simulink model "MicroADAPCPU1"  (R2024a)
settings: Solver=FixedStepAuto  StartTime=0.0  StopTime=Inf  RelTol=1e-3  EnableMultiTasking=on
PreLoadFcn:
  | %Condiciones iniciales
  | id0=single(0);
  | iq0=single(0);
  | w0=single(0);
  | Thetha0=single(0);
  | deltars=0;
  | deltaLd=0;
  | deltaLq=0;
  | deltaphi=0;
  | 
  | %Parametros Axel;
  | Rs=single(1.1); %Ohms
  | L=single(0.00372);
  | Ld=L; %Henrry
  | Lq=L; %Henrry
  | Jm=single(0.00023998); %Kg m2
  | Rm=single(0.0006738); %Nm s
  | rm=Rm;
  | phi=single(0.1099); %Wb
  | %0.0582
  | np=single(8);
values from neighbouring files (symbols this model uses):
  target = mcb_SetProcessorDetails('F28379D',PWM_frequency)    [Para_Motor_Micro.m]
  Ts_com = 2*1*Ts    (= 6e-05)    [Para_Motor_Micro.m]
undefined symbols (not defined in the file or in its folder): C28x, CPU1, CPU2, DiscIntNeverNeededParam, Down, GPTRIP1SEL, GPTRIP2SEL, inverter, PWM_Counter_PeriodVel, TZ1, TZ2, Up
libraries: c2802xlib x12, mcbcontrolslib x9, c2837xDlib x8, simulink x4, mcbpositiondecoderlib x3, c280xlib x3, svdutilitieslib x2, eeTransforms x1, c2000lib x1
(part 1 of 2)
settings Model: ExtModeTrigDuration=8  Creator=axel_  LastModifiedBy=axel_
settings SolverCC: AutoInsertRateTranBlk=on
settings OptimizationCC: DefaultParameterBehavior=Inlined  DefaultUnderspecifiedDataType=single  EnhancedBackFolding=on  PassReuseOutputArgsAs=Individual arguments  MaxStackSize=1024  OptimizeBlockOrder=speed  DifferentSizesBufferReuse=on  OptimizationCustomize=off  DenormalBehavior=FlushToZero  EfficientTunableParamExpr=on
settings DebuggingCC: MultiTaskDSMMsg=none  ParameterPrecisionLossMsg=none  ParameterTunabilityLossMsg=error
settings HardwareCC: ProdBitPerChar=16  ProdBitPerInt=16  ProdBitPerPointer=32  ProdBitPerSizeT=32  ProdBitPerPtrDiffT=32  ProdLargestAtomicInteger=Integer  ProdLargestAtomicFloat=None  ProdWordSize=16  ProdHWDeviceType=Texas Instruments->C2000
settings ModelReferenceCC: ModelReferenceNumInstancesAllowed=Single
settings SFSimCC: MATLABDynamicMemAlloc=off
settings RTWCC: Description=Embedded Coder  SystemTargetFile=ert.tlc  HardwareBoard=TI Delfino F2837xD  TemplateMakefile=ert_default_tmf  Toolchain=Texas Instruments Code Composer Studio (C2000)  GPUComputeCapability=3.5
settings CodeAppCC: ForceParamTrailComments=on  IgnoreCustomStorageClasses=off  OperatorAnnotations=on  SimulinkDataObjDesc=on  SFDataObjDesc=on  InsertBlockDesc=on
settings ERTTargetCC: CodeReplacementLibrary=TI C28x  ExtModeTransport=4  ExtModeStaticAlloc=on  ExtModeAutomaticAllocSize=off  ExtModeStaticAllocSize=10000  ExtModeMexFile=ext_xcp  ExtModeIntrfLevel=Level2 - Open  InlinedParameterPlacement=NonHierarchical

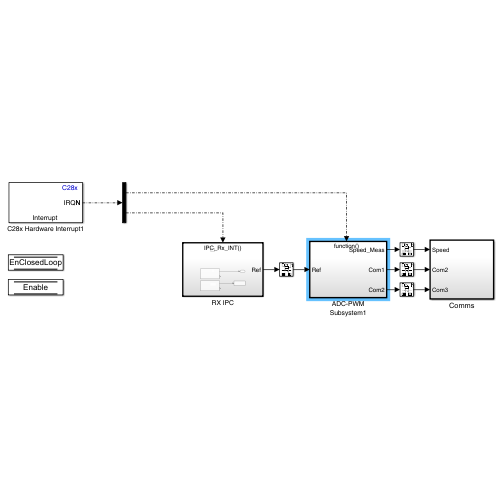
[thumbnail: Simulink's stored preview of the top-level diagram]
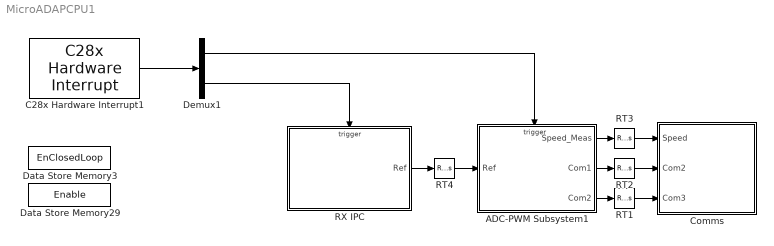
== system MicroADAPCPU1 ==
  ADC-PWM Subsystem1 : Subsystem  TreatAsAtomicUnit=on
  C28x Hardware Interrupt1 : c2000lib/Scheduling/C28x Hardware Interrupt  irqnumbers=[1 1 ]  pienumbers=[1 15 ]  irqpriorities=[30 40 ]  irqpreempts="[1   0  ]"  showinput=off  dspchiptype=C280X
  Comms : Subsystem  TreatAsAtomicUnit=on  SystemSampleTime=Ts_com
  Data Store Memory29 : DataStoreMemory  DataStoreName=Enable  ShowAdditionalParam=off  OutDataTypeStr=boolean
  Data Store Memory3 : DataStoreMemory  DataStoreName=EnClosedLoop  ShowAdditionalParam=off  OutDataTypeStr=boolean
  Demux1 : Demux  Outputs=2
  RT{1..4} (4 alike) : RateTransition  Deterministic=off
  RX IPC : Subsystem
  wires:
  C28x Hardware Interrupt1/1 -> Demux1/1
  Demux1/1 -> ADC-PWM Subsystem1/Trigger
  ADC-PWM Subsystem1/1(Speed_Meas) -> RT3/1
  ADC-PWM Subsystem1/2(Com1) -> RT2/1
  ADC-PWM Subsystem1/3(Com2) -> RT1/1
  RT3/1 -> Comms/1(Speed)
  RT2/1 -> Comms/2(Com2)
  RT1/1 -> Comms/3(Com3)
  RX IPC/1(Ref) -> RT4/1
  Demux1/2 -> RX IPC/Trigger
  RT4/1 -> ADC-PWM Subsystem1/1(Ref)

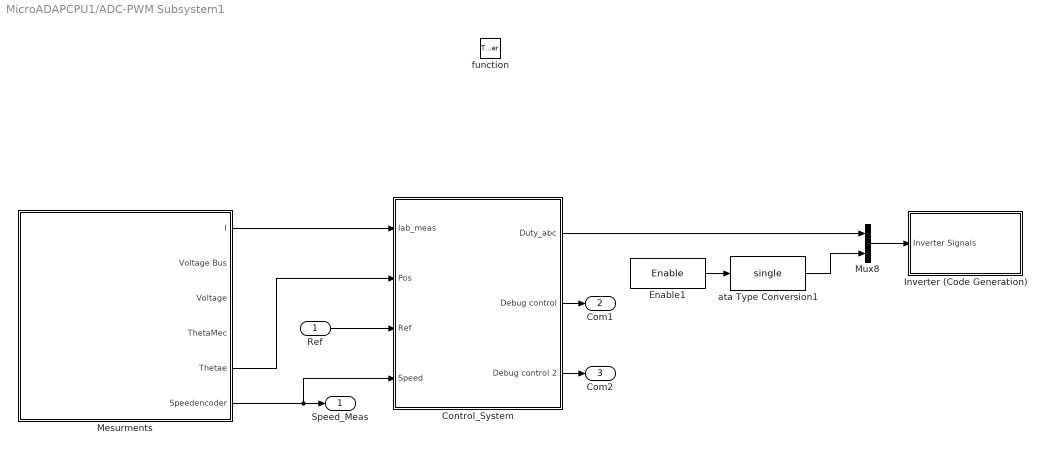
== system MicroADAPCPU1/ADC-PWM Subsystem1 ==
  Ref : Inport
  function : TriggerPort  TriggerType=function-call  VariantControl=Variant  OutputDataType=int8
  Control_System : Subsystem  SystemSampleTime=5e-5
  Enable1 : DataStoreRead  DataStoreName=Enable  IndexOptions=Index vector (dialog)  Indices=1  OutputSizes=1
  Inverter (Code Generation) : Subsystem
  Mesurments : Subsystem
  Mux8 : Mux  Inputs=2
  ata Type Conversion1 : DataTypeConversion  OutDataTypeStr=single  SaturateOnIntegerOverflow=off  RndMeth=Floor
  Speed_Meas : Outport
  Com1 : Outport  Port=2
  Com2 : Outport  Port=3
  wires:
  Ref/1 -> Control_System/3(Ref)
  Mesurments/1(I) -> Control_System/1(Iab_meas)
  Mesurments/6(Speedencoder) -> Control_System/4(Speed), Speed_Meas/1
  Mesurments/5(Thetae) -> Control_System/2(Pos)
  ata Type Conversion1/1 -> Mux8/2
  Control_System/1(Duty_abc) -> Mux8/1
  Enable1/1 -> ata Type Conversion1/1
  Mux8/1 -> Inverter (Code Generation)/1(Inverter Signals)
  Control_System/2(Debug control) -> Com1/1
  Control_System/3(Debug control 2) -> Com2/1

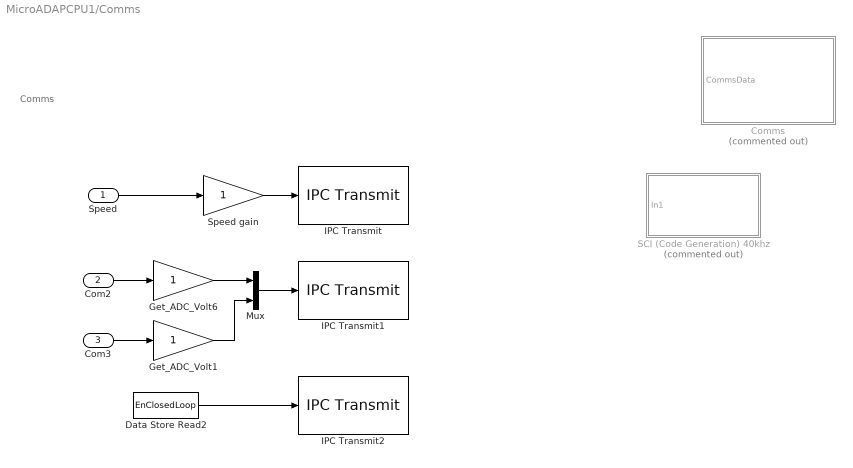
== system MicroADAPCPU1/Comms ==
  note: Comms
  Speed : Inport
  Com2 : Inport  Port=2
  Com3 : Inport  Port=3
  Comms : Subsystem  Commented=on  SystemSampleTime=5e-5
  Data Store Read2 : DataStoreRead  DataStoreName=EnClosedLoop  IndexOptions=Index vector (dialog)  Indices=1  OutputSizes=1
  Get_ADC_Volt1 : Gain  OutDataTypeStr=single  RndMeth=Simplest
  Get_ADC_Volt6 : Gain  OutDataTypeStr=single  RndMeth=Simplest
  IPC Transmit : c2837xDlib/IPC Transmit  blkParamProc=F2837x  SelectDestination=C28x (CPU1/CPU2)  SelectChannel=0  EnableBlocking=off
  IPC Transmit1 : c2837xDlib/IPC Transmit  blkParamProc=F2837x  SelectDestination=C28x (CPU1/CPU2)  SelectChannel=1  EnableBlocking=off
  IPC Transmit2 : c2837xDlib/IPC Transmit  blkParamProc=F2837x  SelectDestination=C28x (CPU1/CPU2)  SelectChannel=4  EnableBlocking=off
  Mux : Mux  Inputs=2
  SCI (Code Generation) 40khz : Subsystem  Commented=on
  Speed gain : Gain  OutDataTypeStr=single  RndMeth=Simplest
  wires:
  Speed/1 -> Speed gain/1
  Com2/1 -> Get_ADC_Volt6/1
  Speed gain/1 -> IPC Transmit/1
  Com3/1 -> Get_ADC_Volt1/1
  Get_ADC_Volt6/1 -> Mux/1
  Get_ADC_Volt1/1 -> Mux/2
  Mux/1 -> IPC Transmit1/1
  Data Store Read2/1 -> IPC Transmit2/1

== system MicroADAPCPU1/RX IPC ==
  note: Data 1
  note: Te
  IPC_Rx_INT : TriggerPort  TriggerType=function-call  VariantControl=Variant
  Data Store Write : DataStoreWrite  DataStoreName=Enable  IndexOptions=Index vector (dialog)  Indices=1  OutputSizes=1
  IPC Receive1 : c2837xDlib/IPC Receive  blkParamProc=F2837x  SelectSource=C28x (CPU1/CPU2)  SelectChannel=2  DataType=single  DataLength=1  EnableBlocking=off  SampleTime=-1
  IPC Receive2 : c2837xDlib/IPC Receive  blkParamProc=F2837x  SelectSource=C28x (CPU1/CPU2)  SelectChannel=3  DataType=boolean  DataLength=1  EnableBlocking=off  SampleTime=-1
  Ref : Outport
  wires:
  IPC Receive1/1 -> Ref/1
  IPC Receive2/1 -> Data Store Write/1

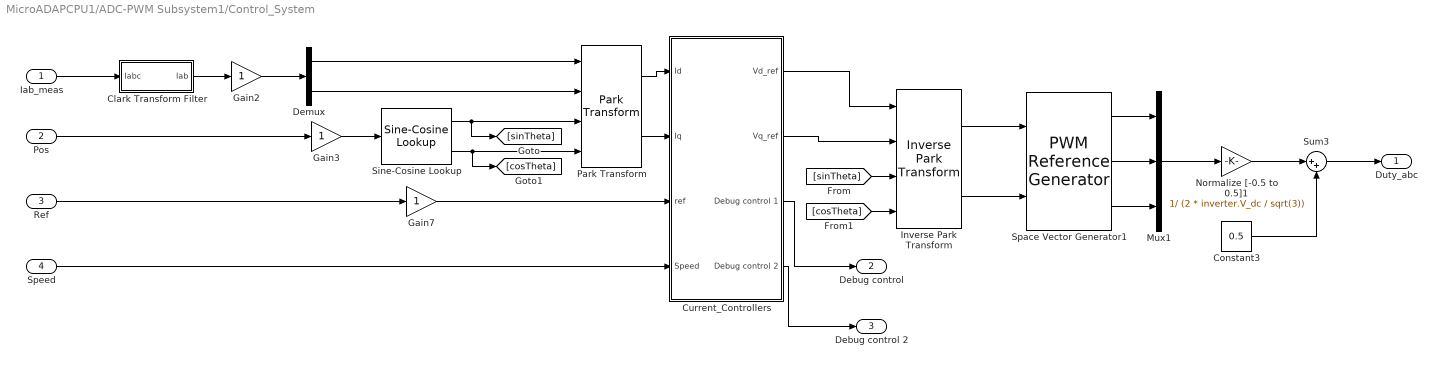
== system MicroADAPCPU1/ADC-PWM Subsystem1/Control_System ==
  Iab_meas : Inport
  Pos : Inport  Port=2
  Ref : Inport  Port=3
  Speed : Inport  Port=4
  Clark Transform Filter : Subsystem
  Constant3 : Constant  Value=0.5  OutDataTypeStr=dataType  SampleTime=-1
  Current_Controllers : Subsystem
  Demux : Demux  Outputs=2
  Gain2 : Gain  OutDataTypeStr=single
  Gain3 : Gain  OutDataTypeStr=single
  Gain7 : Gain
  Inverse Park Transform : mcbcontrolslib/Inverse Park Transform  PhaseInput=Two inputs  AxisAlignment=D-axis  ThetaInput=Sine and Cosine electrical position  AngleInput=Per-unit  N_points=1024
  Mux1 : Mux  Inputs=3
  Normalize [-0.5 to 0.5]1 : Gain  Gain=1/ (2 * inverter.V_dc / sqrt(3))  RndMeth=Simplest  OutDataTypeStr=Inherit: Same as input
  Park Transform : mcbcontrolslib/Park Transform  PhaseInput=Two inputs  AxisAlignment=D-axis  ThetaInput=Sine and Cosine electrical position  AngleInput=Per-unit  N_points=1024
  Sine-Cosine Lookup : mcbcontrolslib/Sine-Cosine Lookup  AngleInput=Radians  N_points=1024  DatatypeInput=Inherit from input  Datatype=single
  Space Vector Generator1 : mcbcontrolslib/PWM Reference Generator  inSignal=Valphabeta  modType=SPWM: sinusoidal PWM
  Sum3 : Sum  Inputs=|++
  Duty_abc : Outport  VectorParamsAs1DForOutWhenUnconnected=off
  Debug control : Outport  Port=2
  Debug control 2 : Outport  Port=3
  wires:
  Gain3/1 -> Sine-Cosine Lookup/1
  Ref/1 -> Gain7/1
  Sine-Cosine Lookup/2 -> Park Transform/4, [cosTheta]
  Park Transform/1 -> Current_Controllers/1(Id)
  Gain2/1 -> Demux/1
  Demux/1 -> Park Transform/1
  Current_Controllers/2(Vq_ref) -> Inverse Park Transform/2
  Pos/1 -> Gain3/1
  [sinTheta] -> Inverse Park Transform/3
  Park Transform/2 -> Current_Controllers/2(Iq)
  Gain7/1 -> Current_Controllers/3(ref)
  [cosTheta] -> Inverse Park Transform/4
  Inverse Park Transform/1 -> Space Vector Generator1/1
  Inverse Park Transform/2 -> Space Vector Generator1/2
  Current_Controllers/1(Vd_ref) -> Inverse Park Transform/1
  Demux/2 -> Park Transform/2
  Sine-Cosine Lookup/1 -> [sinTheta], Park Transform/3
  Speed/1 -> Current_Controllers/4(Speed)
  Space Vector Generator1/3 -> Mux1/3
  Mux1/1 -> Normalize [-0.5 to 0.5]1/1
  Normalize [-0.5 to 0.5]1/1 -> Sum3/1
  Space Vector Generator1/1 -> Mux1/1
  Space Vector Generator1/2 -> Mux1/2
  Constant3/1 -> Sum3/2
  Sum3/1 -> Duty_abc/1
  Iab_meas/1 -> Clark Transform Filter/1(Iabc)
  Clark Transform Filter/1(Iab) -> Gain2/1
  Current_Controllers/3(Debug control 1) -> Debug control/1
  Current_Controllers/4(Debug control 2) -> Debug control 2/1

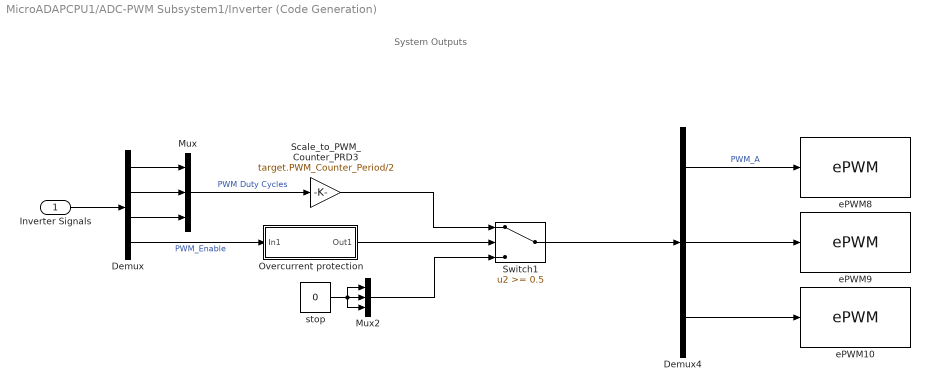
== system MicroADAPCPU1/ADC-PWM Subsystem1/Inverter (Code Generation) ==
  note: System Outputs
  Inverter Signals : Inport
  Demux : Demux
  Demux4 : Demux  Outputs=3
  Mux : Mux  Inputs=3
  Mux2 : Mux  Inputs=3
  Overcurrent protection : Subsystem
  Scale_to_PWM_Counter_PRD3 : Gain  Gain=target.PWM_Counter_Period/2  OutDataTypeStr=uint16  RndMeth=Simplest
  Switch1 : Switch  Threshold=0.5  SaturateOnIntegerOverflow=off  InputSameDT=off
  ePWM10 : c2802xlib/ePWM  PwmType=C2000_Type4  useModule=ePWM3  ePWMxLINKTBPRD=Not Linked  periodUnits=Clock cycles  timerSource=Specify via dialog  timerPeriod_clk=target.PWM_Counter_Period/2+1  timerPeriod_sec=0.0001  tbshadow=Counter equals to zero  countingMode=Up-Down  phaseActiveEnable=Set counter to phase value specified via dialog  phaseDirection=Count up after sync  phaseActive=0  synchronizationEnable=off  dcaevt1Sync=off  dcbevt1Sync=off  synchronizationOption=Pass through (EPWMxSYNCI or SWFSYNC)  dcbevt1SyncOut=off  dcaevt1SyncOut=off  cmpdSyncOut=off  cmpcSyncOut=off  cmpbSyncOut=off  zeroSyncOut=off  swfSyncOut=on  perSynchronizationOption=Counter equals to period (CTR=PRD)  clockPrescale=1  HSclockPrescale=1  enswap=off  ePWMxAStatus=on  ePWMxAactionLogic1=Do nothing  ePWMxAactionLogic2=Do nothing  ePWMxAactionLogic3=Clear  ePWMxAactionLogic4=Set  ePWMxAactionLogic5=Do nothing  ePWMxAactionLogic6=Do nothing  ePWMxACSFenable=off  ePWMxACSFvalue=Forcing disable  ePWMxASFreload=Zero  ePWMxBStatus=off  ePWMxBactionLogic1=Set  ePWMxBactionLogic2=Clear  ePWMxBactionLogic3=Do nothing  ePWMxBactionLogic4=Do nothing  ePWMxBactionLogic5=Clear  ePWMxBactionLogic6=Set  ePWMxBCSFenable=off  ePWMxBCSFvalue=Forcing disable  ePWMxBSFreload=Zero  ePWNxBOutWay=off  ePWMxLINKCMPA=Not Linked  CMPAUnits=Clock cycles  CMPASource=Input port  CMPAValue_per=50  CMPAValue_clk=floor(target.PWM_Counter_Period/4+1)  enCMPAshadow=Counter equals to zero (CTR=Zero)  ePWMxLINKCMPB=Not Linked  CMPBUnits=Clock cycles  CMPBSource=Specify via dialog  CMPBValue_per=50  CMPBValue_clk=floor(target.PWM_Counter_Period/4+1)  enCMPBshadow=Counter equals to zero (CTR=Zero)  ePWMxLINKCMPC=Not Linked  CMPCUnits=Clock cycles  CMPCSource=Specify via dialog  CMPCValue_per=50  CMPCValue_clk=32000  enCMPCshadow=Counter equals to zero (CTR=Zero)  ePWMxLINKCMPD=Not Linked  CMPDUnits=Clock cycles  CMPDSource=Specify via dialog  CMPDValue_per=50  CMPDValue_clk=32000  enCMPDshadow=Counter equals to zero (CTR=Zero)  enableDBePWMxA=on  enableDBePWMxB=on  enhalfcycle=off  DBpolarity=Active high complementary (AHC)  DBedgeDelay=Positive  DBSource_ePWMxA=ePWMxA  DBSource_ePWMxB=ePWMxA  DBPeriodUnits=Clock cycles  DBperiodSource=Specify via dialog  REDperiod=15  FEDperiod=15  REDperiod_sec=0  FEDperiod_sec=0  LoadModeDBRED=Immediate without using shadow  LoadModeDBFED=Immediate without using shadow  adcstartModuleA=off  adcrequestEventA=First event  adcstartEventA=Digital Compare Module A Event 1 start of conversion (DCAEVT1.soc)  adcstartEventA_type2=Counter equals to period (CTR=PRD)  adcstartModuleB=off  adcrequestEventB=First event  adcstartEventB=Counter equals to zero (CTR=Zero)  adcstartEventB_type2=Counter equals to zero (CTR=Zero)  intEn=off  intPrd=First event  intSel=Counter equals to zero (CTR=Zero)  intSel_type2=Counter equals to zero (CTR=Zero)  hrpe=off  enHRPWM=off  HRPWM_LoadMode=Counter equals to period (CTR=PRD)  HRPWM_CTLMode=Duty or Period control mode  HRPWM_EDGMode=Both edge  hrpeb=off  enHRPWMB=off  HRPWM_LoadModeB=Counter equals to zero (CTR=ZERO)  HRPWM_CTLModeB=Duty or Period control mode  HRPWM_EDGModeB=Both edge  enHRDBRED=off  enHRDBFED=off  enSFO=on  enautoconv=on  chopperEnable=off  chopperFrequency=1  chopperFirstwidth=1  chopperDuty=12.5%  tripZonesource=Specify via dialog  tzselOSHT1=off  tzselOSHT2=off  tzselOSHT3=off  tzselOSHT4=off  tzselOSHT5=off  tzselOSHT6=off  tzselOSHDCAEV1=off  tzselOSHDCBEV1=off  tzselCBC1=off  tzselCBC2=off  tzselCBC3=off  tzselCBC4=off  tzselCBC5=off  tzselCBC6=off  tzselCBCDCAEV2=off  tzselCBCDCBEV2=off  enTzOstIntr=off  enTzCbcIntr=off  enTzDCAEVT1Intr=off  enTzDCAEVT2Intr=off  enTzDCBEVT1Intr=off  enTzDCBEVT2Intr=off  tzclrCBCLatch=Counter equals to zero (CTR=Zero)  ePWMxAforced=No action  ePWMxBforced=No action  DCAEVT1forced=No action  DCBEVT1forced=No action  DCAEVT2forced=No action  DCBEVT2forced=No action  dcah=Trip Zone 1 input (TZ1)  dcal=Trip Zone 2 input (TZ2)  dcbh=Trip Zone 1 input (TZ1)  dcbl=Trip Zone 2 input (TZ2)  dcah_type2=GPTRIP1SEL/(TZ1)  dcal_type2=GPTRIP2SEL/(TZ2)  dcbh_type2=GPTRIP1SEL/(TZ1)  dcbl_type2=GPTRIP2SEL/(TZ2)  gendcaevt1=Event disabled  gendcaevt2=Event disabled  gendcbevt1=Event disabled  gendcbevt2=Event disabled  dcaevt1src=DCAEVT1 with sync  dcaevt2src=DCAEVT2 with sync  dcbevt1src=DCBEVT1 with sync  dcbevt2src=DCBEVT2 with sync  pulsesel=Counter equals to zero (CTR=Zero)  blankinv=off  blankoffset=0  blankwidth=0  evsrcsel=Filtered version of DCAEVT1 (DCAEVT1FILT)  encape=off
  ePWM8 : c2802xlib/ePWM  PwmType=C2000_Type4  useModule=ePWM1  ePWMxLINKTBPRD=Not Linked  periodUnits=Clock cycles  timerSource=Specify via dialog  timerPeriod_clk=target.PWM_Counter_Period/2+1  timerPeriod_sec=0.0001  tbshadow=Counter equals to zero  countingMode=Up-Down  phaseActiveEnable=Disable  phaseDirection=Count down after sync  phaseActive=0  synchronizationEnable=off  dcaevt1Sync=off  dcbevt1Sync=off  synchronizationOption=Counter equals to zero (CTR=Zero)  dcbevt1SyncOut=off  dcaevt1SyncOut=off  cmpdSyncOut=off  cmpcSyncOut=off  cmpbSyncOut=off  zeroSyncOut=on  swfSyncOut=off  perSynchronizationOption=Counter equals to period (CTR=PRD)  clockPrescale=1  HSclockPrescale=1  enswap=off  ePWMxAStatus=on  ePWMxAactionLogic1=Do nothing  ePWMxAactionLogic2=Do nothing  ePWMxAactionLogic3=Clear  ePWMxAactionLogic4=Set  ePWMxAactionLogic5=Do nothing  ePWMxAactionLogic6=Do nothing  ePWMxACSFenable=off  ePWMxACSFvalue=Forcing disable  ePWMxASFreload=Zero  ePWMxBStatus=off  ePWMxBactionLogic1=Set  ePWMxBactionLogic2=Clear  ePWMxBactionLogic3=Do nothing  ePWMxBactionLogic4=Do nothing  ePWMxBactionLogic5=Clear  ePWMxBactionLogic6=Set  ePWMxBCSFenable=off  ePWMxBCSFvalue=Forcing disable  ePWMxBSFreload=Zero  ePWNxBOutWay=off  ePWMxLINKCMPA=Not Linked  CMPAUnits=Clock cycles  CMPASource=Input port  CMPAValue_per=50  CMPAValue_clk=floor(target.PWM_Counter_Period/4+1)  enCMPAshadow=Counter equals to zero (CTR=Zero)  ePWMxLINKCMPB=Not Linked  CMPBUnits=Clock cycles  CMPBSource=Specify via dialog  CMPBValue_per=50  CMPBValue_clk=floor(target.PWM_Counter_Period/4+1)  enCMPBshadow=Counter equals to zero (CTR=Zero)  ePWMxLINKCMPC=Not Linked  CMPCUnits=Clock cycles  CMPCSource=Specify via dialog  CMPCValue_per=50  CMPCValue_clk=32000  enCMPCshadow=Counter equals to zero (CTR=Zero)  ePWMxLINKCMPD=Not Linked  CMPDUnits=Clock cycles  CMPDSource=Specify via dialog  CMPDValue_per=50  CMPDValue_clk=32000  enCMPDshadow=Counter equals to zero (CTR=Zero)  enableDBePWMxA=on  enableDBePWMxB=on  enhalfcycle=off  DBpolarity=Active high complementary (AHC)  DBedgeDelay=Positive  DBSource_ePWMxA=ePWMxA  DBSource_ePWMxB=ePWMxA  DBPeriodUnits=Clock cycles  DBperiodSource=Specify via dialog  REDperiod=15  FEDperiod=15  REDperiod_sec=0  FEDperiod_sec=0  LoadModeDBRED=Immediate without using shadow  LoadModeDBFED=Immediate without using shadow  adcstartModuleA=on  adcrequestEventA=First event  adcstartEventA=Digital Compare Module A Event 1 start of conversion (DCAEVT1.soc)  adcstartEventA_type2=Counter equals to period (CTR=PRD)  adcstartModuleB=off  adcrequestEventB=First event  adcstartEventB=Counter equals to zero (CTR=Zero)  adcstartEventB_type2=Counter equals to zero (CTR=Zero)  intEn=on  intPrd=First event  intSel=Counter equals to zero (CTR=Zero)  intSel_type2=Counter equals to period (CTR=PRD)  hrpe=off  enHRPWM=off  HRPWM_LoadMode=Counter equals to period (CTR=PRD)  HRPWM_CTLMode=Duty or Period control mode  HRPWM_EDGMode=Both edge  hrpeb=off  enHRPWMB=off  HRPWM_LoadModeB=Counter equals to zero (CTR=ZERO)  HRPWM_CTLModeB=Duty or Period control mode  HRPWM_EDGModeB=Both edge  enHRDBRED=off  enHRDBFED=off  enSFO=on  enautoconv=on  chopperEnable=off  chopperFrequency=1  chopperFirstwidth=1  chopperDuty=12.5%  tripZonesource=Specify via dialog  tzselOSHT1=off  tzselOSHT2=off  tzselOSHT3=off  tzselOSHT4=off  tzselOSHT5=off  tzselOSHT6=off  tzselOSHDCAEV1=off  tzselOSHDCBEV1=off  tzselCBC1=off  tzselCBC2=off  tzselCBC3=off  tzselCBC4=off  tzselCBC5=off  tzselCBC6=off  tzselCBCDCAEV2=off  tzselCBCDCBEV2=off  enTzOstIntr=off  enTzCbcIntr=off  enTzDCAEVT1Intr=off  enTzDCAEVT2Intr=off  enTzDCBEVT1Intr=off  enTzDCBEVT2Intr=off  tzclrCBCLatch=Counter equals to zero (CTR=Zero)  ePWMxAforced=No action  ePWMxBforced=No action  DCAEVT1forced=No action  DCBEVT1forced=No action  DCAEVT2forced=No action  DCBEVT2forced=No action  dcah=Trip Zone 1 input (TZ1)  dcal=Trip Zone 2 input (TZ2)  dcbh=Trip Zone 1 input (TZ1)  dcbl=Trip Zone 2 input (TZ2)  dcah_type2=GPTRIP1SEL/(TZ1)  dcal_type2=GPTRIP2SEL/(TZ2)  dcbh_type2=GPTRIP1SEL/(TZ1)  dcbl_type2=GPTRIP2SEL/(TZ2)  gendcaevt1=Event disabled  gendcaevt2=Event disabled  gendcbevt1=Event disabled  gendcbevt2=Event disabled  dcaevt1src=DCAEVT1 with sync  dcaevt2src=DCAEVT2 with sync  dcbevt1src=DCBEVT1 with sync  dcbevt2src=DCBEVT2 with sync  pulsesel=Counter equals to zero (CTR=Zero)  blankinv=off  blankoffset=0  blankwidth=0  evsrcsel=Filtered version of DCAEVT1 (DCAEVT1FILT)  encape=off
  ePWM9 : c2802xlib/ePWM  PwmType=C2000_Type4  useModule=ePWM2  ePWMxLINKTBPRD=Not Linked  periodUnits=Clock cycles  timerSource=Specify via dialog  timerPeriod_clk=target.PWM_Counter_Period/2+1  timerPeriod_sec=0.0001  tbshadow=Counter equals to zero  countingMode=Up-Down  phaseActiveEnable=Set counter to phase value specified via dialog  phaseDirection=Count up after sync  phaseActive=0  synchronizationEnable=off  dcaevt1Sync=off  dcbevt1Sync=off  synchronizationOption=Pass through (EPWMxSYNCI or SWFSYNC)  dcbevt1SyncOut=off  dcaevt1SyncOut=off  cmpdSyncOut=off  cmpcSyncOut=off  cmpbSyncOut=off  zeroSyncOut=off  swfSyncOut=on  perSynchronizationOption=Counter equals to period (CTR=PRD)  clockPrescale=1  HSclockPrescale=1  enswap=off  ePWMxAStatus=on  ePWMxAactionLogic1=Do nothing  ePWMxAactionLogic2=Do nothing  ePWMxAactionLogic3=Clear  ePWMxAactionLogic4=Set  ePWMxAactionLogic5=Do nothing  ePWMxAactionLogic6=Do nothing  ePWMxACSFenable=off  ePWMxACSFvalue=Forcing disable  ePWMxASFreload=Zero  ePWMxBStatus=off  ePWMxBactionLogic1=Set  ePWMxBactionLogic2=Clear  ePWMxBactionLogic3=Do nothing  ePWMxBactionLogic4=Do nothing  ePWMxBactionLogic5=Clear  ePWMxBactionLogic6=Set  ePWMxBCSFenable=off  ePWMxBCSFvalue=Forcing disable  ePWMxBSFreload=Zero  ePWNxBOutWay=off  ePWMxLINKCMPA=Not Linked  CMPAUnits=Clock cycles  CMPASource=Input port  CMPAValue_per=50  CMPAValue_clk=floor(target.PWM_Counter_Period/4+1)  enCMPAshadow=Counter equals to zero (CTR=Zero)  ePWMxLINKCMPB=Not Linked  CMPBUnits=Clock cycles  CMPBSource=Specify via dialog  CMPBValue_per=50  CMPBValue_clk=floor(target.PWM_Counter_Period/4+1)  enCMPBshadow=Counter equals to zero (CTR=Zero)  ePWMxLINKCMPC=Not Linked  CMPCUnits=Clock cycles  CMPCSource=Specify via dialog  CMPCValue_per=50  CMPCValue_clk=32000  enCMPCshadow=Counter equals to zero (CTR=Zero)  ePWMxLINKCMPD=Not Linked  CMPDUnits=Clock cycles  CMPDSource=Specify via dialog  CMPDValue_per=50  CMPDValue_clk=32000  enCMPDshadow=Counter equals to zero (CTR=Zero)  enableDBePWMxA=on  enableDBePWMxB=on  enhalfcycle=off  DBpolarity=Active high complementary (AHC)  DBedgeDelay=Positive  DBSource_ePWMxA=ePWMxA  DBSource_ePWMxB=ePWMxA  DBPeriodUnits=Clock cycles  DBperiodSource=Specify via dialog  REDperiod=15  FEDperiod=15  REDperiod_sec=0  FEDperiod_sec=0  LoadModeDBRED=Immediate without using shadow  LoadModeDBFED=Immediate without using shadow  adcstartModuleA=off  adcrequestEventA=First event  adcstartEventA=Digital Compare Module A Event 1 start of conversion (DCAEVT1.soc)  adcstartEventA_type2=Counter equals to period (CTR=PRD)  adcstartModuleB=off  adcrequestEventB=First event  adcstartEventB=Counter equals to zero (CTR=Zero)  adcstartEventB_type2=Counter equals to zero (CTR=Zero)  intEn=off  intPrd=First event  intSel=Counter equals to zero (CTR=Zero)  intSel_type2=Counter equals to zero (CTR=Zero)  hrpe=off  enHRPWM=off  HRPWM_LoadMode=Counter equals to period (CTR=PRD)  HRPWM_CTLMode=Duty or Period control mode  HRPWM_EDGMode=Both edge  hrpeb=off  enHRPWMB=off  HRPWM_LoadModeB=Counter equals to zero (CTR=ZERO)  HRPWM_CTLModeB=Duty or Period control mode  HRPWM_EDGModeB=Both edge  enHRDBRED=off  enHRDBFED=off  enSFO=on  enautoconv=on  chopperEnable=off  chopperFrequency=1  chopperFirstwidth=1  chopperDuty=12.5%  tripZonesource=Specify via dialog  tzselOSHT1=off  tzselOSHT2=off  tzselOSHT3=off  tzselOSHT4=off  tzselOSHT5=off  tzselOSHT6=off  tzselOSHDCAEV1=off  tzselOSHDCBEV1=off  tzselCBC1=off  tzselCBC2=off  tzselCBC3=off  tzselCBC4=off  tzselCBC5=off  tzselCBC6=off  tzselCBCDCAEV2=off  tzselCBCDCBEV2=off  enTzOstIntr=off  enTzCbcIntr=off  enTzDCAEVT1Intr=off  enTzDCAEVT2Intr=off  enTzDCBEVT1Intr=off  enTzDCBEVT2Intr=off  tzclrCBCLatch=Counter equals to zero (CTR=Zero)  ePWMxAforced=No action  ePWMxBforced=No action  DCAEVT1forced=No action  DCBEVT1forced=No action  DCAEVT2forced=No action  DCBEVT2forced=No action  dcah=Trip Zone 1 input (TZ1)  dcal=Trip Zone 2 input (TZ2)  dcbh=Trip Zone 1 input (TZ1)  dcbl=Trip Zone 2 input (TZ2)  dcah_type2=GPTRIP1SEL/(TZ1)  dcal_type2=GPTRIP2SEL/(TZ2)  dcbh_type2=GPTRIP1SEL/(TZ1)  dcbl_type2=GPTRIP2SEL/(TZ2)  gendcaevt1=Event disabled  gendcaevt2=Event disabled  gendcbevt1=Event disabled  gendcbevt2=Event disabled  dcaevt1src=DCAEVT1 with sync  dcaevt2src=DCAEVT2 with sync  dcbevt1src=DCBEVT1 with sync  dcbevt2src=DCBEVT2 with sync  pulsesel=Counter equals to zero (CTR=Zero)  blankinv=off  blankoffset=0  blankwidth=0  evsrcsel=Filtered version of DCAEVT1 (DCAEVT1FILT)  encape=off
  stop : Constant  Value=0  OutDataTypeStr=uint16
  wires:
  Scale_to_PWM_Counter_PRD3/1 -> Switch1/1
  Mux2/1 -> Switch1/3
  stop/1 -> Mux2/3, Mux2/2, Mux2/1
  Demux/4 -> Overcurrent protection/1(In1)  "PWM_Enable"
  Inverter Signals/1 -> Demux/1
  Mux/1 -> Scale_to_PWM_Counter_PRD3/1  "PWM Duty Cycles"
  Demux/1 -> Mux/1
  Demux/2 -> Mux/2
  Demux/3 -> Mux/3
  Overcurrent protection/1(Out1) -> Switch1/2
  Demux4/3 -> ePWM10/1
  Demux4/1 -> ePWM8/1  "PWM_A"
  Switch1/1 -> Demux4/1
  Demux4/2 -> ePWM9/1

== system MicroADAPCPU1/ADC-PWM Subsystem1/Mesurments ==
  Current mesurment : Subsystem
  Position Mesurment : Subsystem
  Voltage Mesurment : Subsystem
  I : Outport
  Voltage Bus : Outport  Port=2
  Voltage : Outport  Port=3
  ThetaMec : Outport  Port=4
  Thetae : Outport  Port=5
  Speedencoder : Outport  Port=6
  wires:
  Current mesurment/1(Out1) -> I/1
  Voltage Mesurment/1(Out1) -> Voltage Bus/1
  Voltage Mesurment/2(Vol) -> Voltage/1
  Position Mesurment/1(ThetaE) -> Thetae/1
  Position Mesurment/3(ThetaMec) -> ThetaMec/1
  Position Mesurment/2(speedfb) -> Speedencoder/1

== system MicroADAPCPU1/Comms/Comms ==
  CommsData : Inport
  SCI (Serial Comunication) : Subsystem
  Selector : Selector  InputPortWidth=2  IndexOptions=Index vector (port)  Indices=[1 3]  OutputSizes=1
  speed_control : Constant  Value=[1 2]  OutDataTypeStr=uint16  SampleTime=-1
  wires:
  Selector/1 -> SCI (Serial Comunication)/1(In1)
  CommsData/1 -> Selector/1
  speed_control/1 -> Selector/2

== system MicroADAPCPU1/Comms/SCI (Code Generation) 40khz ==
  In1 : Inport
  Byte Pack : svdutilitieslib/Byte Pack  maskPackedDataType=uint32  datatypes={'single'}  byteAlign=4  blockPlatform=tic2000
  Data_Logging : Subsystem
  Demux2 : Demux  Outputs=2
  While Iterator Subsystem : Subsystem  TreatAsAtomicUnit=on
  wires:
  Byte Pack/1 -> Data_Logging/1(Data_Log)
  Data_Logging/1(SCI_Tx) -> Demux2/1
  In1/1 -> Byte Pack/1
  Demux2/1 -> While Iterator Subsystem/1(Data)  "SCI_Tx_Data"
  Demux2/2 -> While Iterator Subsystem/2(Iteration)  "SCI_Tx_Iteration"

== system MicroADAPCPU1/ADC-PWM Subsystem1/Control_System/Clark Transform Filter ==
  Iabc : Inport
  Add : Sum  Inputs=--
  Clarke Transformation : Subsystem  Commented=through  InitFcn=tic2000lib_licenseCheck  mask(Clarke Transformation){}
      mask help: This block performs transformation of three-phase quantities into balanced two-phase quadrature quantities. All inputs and outputs are signed 32-bit fixed-point numbers with Q value between 1 and 29.
      mask Help: eval('linkfoundation.util.openBlockHelp(''c28xdmclibclarketransformation'',''ecoder'')');
      mask Display:
      | port_label('input',1,'As');
      | port_label('input',2,'Bs');
      | port_label('Output',1,'Alpha');
      | port_label('Output',2,'Beta');
      | text(0.5,0.15, 'Clarke', 'horizontalalignment','center');
  Clarke Transform : eeTransforms/Clarke Transform  PowerInvariant=off
      settings: LibrarySourceBlock=|
      | ee_sl_lib/Mathematical
      | Transforms/Clarke Transform
  Demux : Demux  Outputs=3
  Demux1 : Demux  Outputs=3
  Mux : Mux  Inputs=3
  Mux1 : Mux  Inputs=2
  Iab : Outport
  wires:
  Iabc/1 -> Demux/1
  Demux/2 -> Mux/2, Add/2
  Demux/1 -> Mux/1, Add/1
  Mux1/1 -> Iab/1
  Add/1 -> Mux/3
  Mux/1 -> Clarke Transform/1
  Clarke Transform/1 -> Demux1/1
  Demux1/1 -> Mux1/1
  Demux1/2 -> Mux1/2

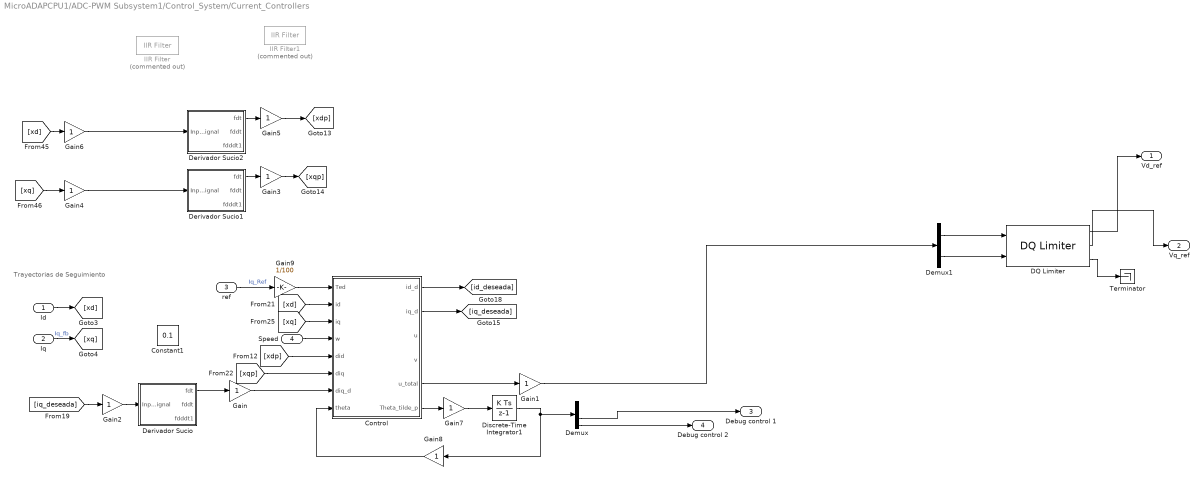
== system MicroADAPCPU1/ADC-PWM Subsystem1/Control_System/Current_Controllers ==
  note: Trayectorias de Seguimiento
  Id : Inport
  Iq : Inport  Port=2
  ref : Inport  Port=3
  Speed : Inport  Port=4
  Constant1 : Constant  Value=0.1  OutDataTypeStr=single
  "Control " : MATLAB Function  TreatAsAtomicUnit=on
  DQ Limiter : mcbcontrolslib/DQ Limiter  satMethodInputType=Specify via dialog  satMethodSelected=D-Q equivalence  satLimitInputType=Specify via dialog  Vmax=inverter.V_dc/sqrt(3) *1
  Demux : Demux
  Demux1 : Demux  Outputs=2
  Derivador Sucio : Subsystem  mask{L=100}
      mask prompts: L "Ganacia de los Filtros"
      mask DialogControl DescTextVar Prompt: Derivador Sucio
  Derivador Sucio1 : Subsystem  mask{L=100}
      mask prompts: L "Ganacia de los Filtros"
      mask DialogControl DescTextVar Prompt: Derivador Sucio
  Derivador Sucio2 : Subsystem  mask{L=100}
      mask prompts: L "Ganacia de los Filtros"
      mask DialogControl DescTextVar Prompt: Derivador Sucio
  Discrete-Time Integrator1 : DiscreteIntegrator  InitialCondition=[deltars; deltaLd; deltaLq; deltaphi]  SampleTime=-1  ICPrevOutput=DiscIntNeverNeededParam  ICPrevScaledInput=DiscIntNeverNeededParam
  Gain{,1,3,5,8} (5 alike) : Gain  OutDataTypeStr=single
  Gain{2,4,6..7} (4 alike) : Gain  OutDataTypeStr=double
  Gain9 : Gain  Gain=1/100  OutDataTypeStr=double
  IIR Filter : mcbcontrolslib/IIR Filter  Commented=on  VariantControl=Low Pass Filter  VariantSelect=Low-pass  FilterConstantInputType=Specify via dialog  Filter_constant=0.04  advancedSettings=on  Ts=5e-5  cutOff_freq=132.6291
  IIR Filter1 : mcbcontrolslib/IIR Filter  Commented=on  VariantControl=Low Pass Filter  VariantSelect=Low-pass  FilterConstantInputType=Specify via dialog  Filter_constant=0.01  advancedSettings=off  Ts=10e-6  cutOff_freq=160.7626
  Terminator : Terminator
  Vd_ref : Outport  VectorParamsAs1DForOutWhenUnconnected=off
  Vq_ref : Outport  Port=2  VectorParamsAs1DForOutWhenUnconnected=off
  Debug control 1 : Outport  Port=3
  Debug control 2 : Outport  Port=4
  wires:
  DQ Limiter/2 -> Vq_ref/1
  DQ Limiter/1 -> Vd_ref/1
  DQ Limiter/3 -> Terminator/1
  Gain1/1 -> Demux1/1
  Demux1/1 -> DQ Limiter/1
  Demux1/2 -> DQ Limiter/2
  Gain5/1 -> [xdp]
  [xd] -> Gain6/1
  [xq] -> Gain4/1
  Id/1 -> [xd]
  Iq/1 -> [xq]  "Iq_fb"
  [xqp] -> "Control "/6(diq)
  [xdp] -> "Control "/5(did)
  [iq_deseada] -> Gain2/1
  "Control "/1(id_d) -> [id_deseada]
  [xq] -> "Control "/3(iq)
  Speed/1 -> "Control "/4(w)
  [xd] -> "Control "/2(id)
  "Control "/6(Theta_tilde_p) -> Gain7/1
  Gain/1 -> "Control "/7(diq_d)
  Derivador Sucio/1(fdt) -> Gain/1
  Gain2/1 -> Derivador Sucio/1(Input Signal)
  Derivador Sucio1/1(fdt) -> Gain3/1
  Derivador Sucio2/1(fdt) -> Gain5/1
  Gain3/1 -> [xqp]
  Gain7/1 -> Discrete-Time Integrator1/1
  Gain8/1 -> "Control "/8(theta)
  ref/1 -> Gain9/1  "Iq_Ref"
  Gain6/1 -> Derivador Sucio2/1(Input Signal)
  Gain4/1 -> Derivador Sucio1/1(Input Signal)
  Discrete-Time Integrator1/1 -> Gain8/1, Demux/1
  Gain9/1 -> "Control "/1(Ted)
  "Control "/5(u_total) -> Gain1/1
  "Control "/2(iq_d) -> [iq_deseada]
  Demux/3 -> Debug control 1/1
  Demux/4 -> Debug control 2/1

== system MicroADAPCPU1/ADC-PWM Subsystem1/Inverter (Code Generation)/Overcurrent protection ==
  In1 : Inport
  AND : Logic  IconShape=distinctive  AllPortsSameDT=off  OutDataTypeStr=boolean
  Digital Input : c2837xDlib/Digital Input  GPIO_Number=GPIO40~GPIO47  GPIO_Bit0=off  GPIO_Bit1=off  GPIO_Bit2=off  GPIO_Bit3=on  GPIO_Bit4=off  GPIO_Bit5=off  GPIO_Bit6=off  GPIO_Bit7=off  sampleTime=-1  dataType=boolean  GPIO_Bit0_Qualification=Sync to SYSCLKOUT  GPIO_Bit1_Qualification=Sync to SYSCLKOUT  GPIO_Bit2_Qualification=Sync to SYSCLKOUT  GPIO_Bit3_Qualification=Sync to SYSCLKOUT  GPIO_Bit4_Qualification=Sync to SYSCLKOUT  GPIO_Bit5_Qualification=Sync to SYSCLKOUT  GPIO_Bit6_Qualification=Sync to SYSCLKOUT  GPIO_Bit7_Qualification=Sync to SYSCLKOUT  Qualification_Period=-1
  Digital Output1 : c2837xDlib/Digital Output  GPIO_Number=GPIO24~GPIO31  GPIO_Bit0=off  GPIO_BIT0_Toggle=on  GPIO_Bit1=off  GPIO_BIT1_Toggle=off  GPIO_Bit2=off  GPIO_BIT2_Toggle=off  GPIO_Bit3=off  GPIO_BIT3_Toggle=off  GPIO_Bit4=off  GPIO_BIT4_Toggle=off  GPIO_Bit5=off  GPIO_BIT5_Toggle=off  GPIO_Bit6=off  GPIO_BIT6_Toggle=off  GPIO_Bit7=on  GPIO_BIT7_Toggle=off
  Digital Output2 : c2837xDlib/Digital Output  GPIO_Number=GPIO8~GPIO15  GPIO_Bit0=off  GPIO_BIT0_Toggle=on  GPIO_Bit1=on  GPIO_BIT1_Toggle=off  GPIO_Bit2=off  GPIO_BIT2_Toggle=off  GPIO_Bit3=off  GPIO_BIT3_Toggle=off  GPIO_Bit4=off  GPIO_BIT4_Toggle=off  GPIO_Bit5=off  GPIO_BIT5_Toggle=off  GPIO_Bit6=off  GPIO_BIT6_Toggle=off  GPIO_Bit7=off  GPIO_BIT7_Toggle=off
  Enable1 : DataStoreRead  DataStoreName=EnClosedLoop  IndexOptions=Index vector (dialog)  Indices=1  OutputSizes=1
  NOT : Logic  Operator=NOT  IconShape=distinctive  AllPortsSameDT=off  OutDataTypeStr=boolean
  ata Type Conversion1 : DataTypeConversion  OutDataTypeStr=dataType  SaturateOnIntegerOverflow=off  RndMeth=Floor
  Out1 : Outport
  wires:
  NOT/1 -> AND/2, Digital Output1/1
  Digital Input/1 -> NOT/1  "PWM_Enable"
  AND/1 -> Out1/1
  In1/1 -> AND/1
  ata Type Conversion1/1 -> Digital Output2/1
  Enable1/1 -> ata Type Conversion1/1

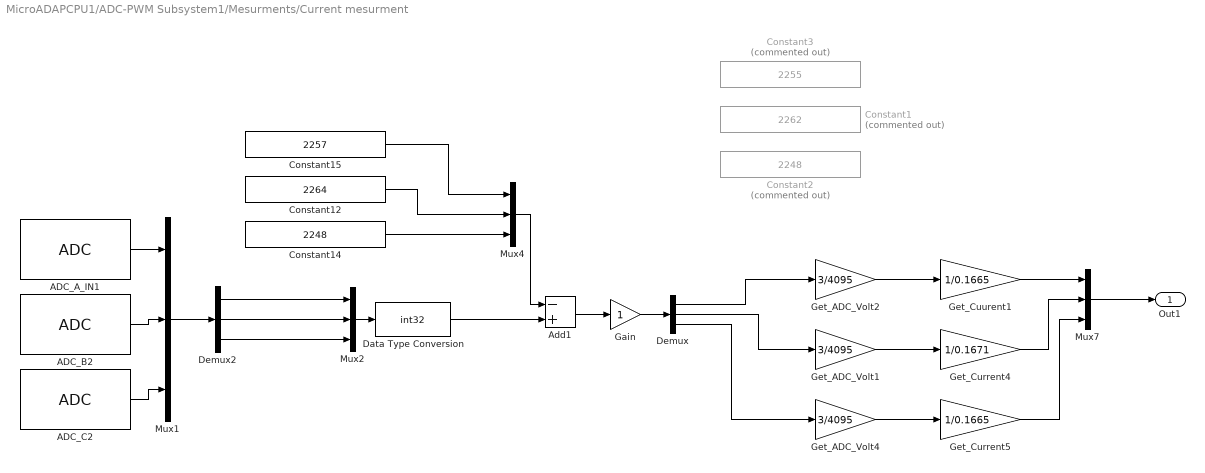
== system MicroADAPCPU1/ADC-PWM Subsystem1/Mesurments/Current mesurment ==
  ADC_A_IN1 : c2802xlib/ADC  blkParamProc=C2000_Type4  ADCModule=B  samplingMode=Single sample mode  ADCResolution=12-bit (Single-ended input)  useSOC1=SOC0  useSOC2=SOC0_SOC1  SOCAcquisitionWindow=15  SOCTriggerSource=ePWM1_ADCSOCA  SOCInterruptTrigger=No ADCINT  Ts=-1  dType=uint16  postInterrupt=off  interruptSel=ADCINT1  ADCINTContinuous=on  endma=off  chdma=1  conv1=ADCINA0  conv2=ADCINA0 and ADCINB0  conv1_Type4=ADCIN3  conv2_Type4=ADCIN0 and ADCIN1
  ADC_B2 : c2802xlib/ADC  blkParamProc=C2000_Type4  ADCModule=B  samplingMode=Single sample mode  ADCResolution=12-bit (Single-ended input)  useSOC1=SOC1  useSOC2=SOC0_SOC1  SOCAcquisitionWindow=15  SOCTriggerSource=ePWM1_ADCSOCA  SOCInterruptTrigger=No ADCINT  Ts=-1  dType=uint16  postInterrupt=off  interruptSel=ADCINT1  ADCINTContinuous=on  endma=off  chdma=1  conv1=ADCINA0  conv2=ADCINA0 and ADCINB0  conv1_Type4=ADCIN5  conv2_Type4=ADCIN0 and ADCIN1
  ADC_C2 : c2802xlib/ADC  blkParamProc=C2000_Type4  ADCModule=A  samplingMode=Single sample mode  ADCResolution=12-bit (Single-ended input)  useSOC1=SOC0  useSOC2=SOC0_SOC1  SOCAcquisitionWindow=15  SOCTriggerSource=ePWM1_ADCSOCA  SOCInterruptTrigger=No ADCINT  Ts=-1  dType=uint16  postInterrupt=on  interruptSel=ADCINT1  ADCINTContinuous=on  endma=off  chdma=1  conv1=ADCINA0  conv2=ADCINA0 and ADCINB0  conv1_Type4=ADCIN5  conv2_Type4=ADCIN0 and ADCIN1
  Add1 : Sum  Inputs=-+
  Constant1 : Constant  Commented=on  Value=2262  OutDataTypeStr=single
  Constant12 : Constant  Value=2264  OutDataTypeStr=single
  Constant14 : Constant  Value=2248  OutDataTypeStr=single
  Constant15 : Constant  Value=2257  OutDataTypeStr=single
  Constant2 : Constant  Commented=on  Value=2248  OutDataTypeStr=single
  Constant3 : Constant  Commented=on  Value=2255  OutDataTypeStr=single
  Data Type Conversion : DataTypeConversion  OutDataTypeStr=int32  ConvertRealWorld=Stored Integer (SI)  RndMeth=Simplest  SaturateOnIntegerOverflow=off
  Demux : Demux  Outputs=3
  Demux2 : Demux  Outputs=3
  Gain : Gain  OutDataTypeStr=single
  Get_ADC_Volt1 : Gain  Gain=3/4095  OutDataTypeStr=single  RndMeth=Simplest
  Get_ADC_Volt2 : Gain  Gain=3/4095  OutDataTypeStr=single  RndMeth=Simplest
  Get_ADC_Volt4 : Gain  Gain=3/4095  OutDataTypeStr=single  RndMeth=Simplest
  Get_Current4 : Gain  Gain=1/0.1671  OutDataTypeStr=single  RndMeth=Simplest
  Get_Current5 : Gain  Gain=1/0.1665  OutDataTypeStr=single  RndMeth=Simplest
  Get_Cuurent1 : Gain  Gain=1/0.1665  OutDataTypeStr=single  RndMeth=Simplest
  Mux{1..2,4,7} (4 alike) : Mux  Inputs=3
  Out1 : Outport
  wires:
  Data Type Conversion/1 -> Add1/2
  ADC_C2/1 -> Mux1/3
  Mux2/1 -> Data Type Conversion/1
  Demux2/2 -> Mux2/2
  Add1/1 -> Gain/1
  Demux2/3 -> Mux2/3
  Mux1/1 -> Demux2/1
  Mux4/1 -> Add1/1
  Demux/1 -> Get_ADC_Volt2/1
  ADC_B2/1 -> Mux1/2
  Demux/2 -> Get_ADC_Volt1/1
  Get_ADC_Volt2/1 -> Get_Cuurent1/1
  ADC_A_IN1/1 -> Mux1/1
  Get_ADC_Volt4/1 -> Get_Current5/1
  Get_ADC_Volt1/1 -> Get_Current4/1
  Demux/3 -> Get_ADC_Volt4/1
  Demux2/1 -> Mux2/1
  Mux7/1 -> Out1/1
  Get_Cuurent1/1 -> Mux7/1
  Get_Current4/1 -> Mux7/2
  Get_Current5/1 -> Mux7/3
  Gain/1 -> Demux/1
  Constant15/1 -> Mux4/1
  Constant12/1 -> Mux4/2
  Constant14/1 -> Mux4/3

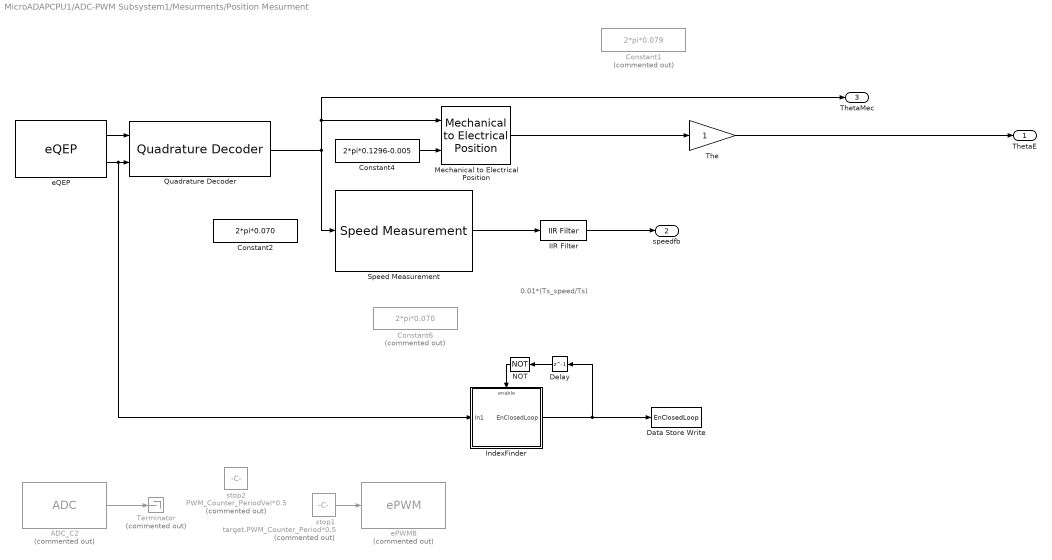
== system MicroADAPCPU1/ADC-PWM Subsystem1/Mesurments/Position Mesurment ==
  note: 0.01*(Ts_speed/Ts)
  ADC_C2 : c2802xlib/ADC  Commented=on  blkParamProc=C2000_Type4  ADCModule=C  samplingMode=Single sample mode  ADCResolution=12-bit (Single-ended input)  useSOC1=SOC5  useSOC2=SOC0_SOC1  SOCAcquisitionWindow=15  SOCTriggerSource=ePWM4_ADCSOCA  SOCInterruptTrigger=No ADCINT  Ts=-1  dType=uint16  postInterrupt=on  interruptSel=ADCINT1  ADCINTContinuous=on  endma=off  chdma=1  conv1=ADCINA0  conv2=ADCINA0 and ADCINB0  conv1_Type4=ADCIN0  conv2_Type4=ADCIN0 and ADCIN1
  Constant1 : Constant  Commented=on  Value=2*pi*0.079  OutDataTypeStr=single
  Constant2 : Constant  Value=2*pi*0.070  OutDataTypeStr=single
  Constant4 : Constant  Value=2*pi*0.1296-0.005  OutDataTypeStr=single
  Constant6 : Constant  Commented=on  Value=2*pi*0.070  OutDataTypeStr=single
  Data Store Write : DataStoreWrite  DataStoreName=EnClosedLoop  IndexOptions=Index vector (dialog)  Indices=1  OutputSizes=1
  Delay : Delay  DelayLength=1
  IIR Filter : mcbcontrolslib/IIR Filter  VariantControl=Low Pass Filter  VariantSelect=Low-pass  FilterConstantInputType=Specify via dialog  Filter_constant=0.01  advancedSettings=off  Ts=10e-6  cutOff_freq=160.7626
  IndexFinder : Subsystem
  Mechanical to Electrical Position : mcbpositiondecoderlib/Mechanical to Electrical Position  PolePairsInputType=Specify via dialog  NrPP=4  selectedRange=Radians  MechOfstInputType=Input port  mechOffsetIn=0  maxAngleIn=2*pi  InputDataType=single  VariantSelect=floating-point
  NOT : Logic  Operator=NOT  AllPortsSameDT=off  OutDataTypeStr=boolean
  Quadrature Decoder : mcbpositiondecoderlib/Quadrature Decoder  EncoderSlitsPerRevolution=2048  EncoderCountsPerSlit=4  CounterSize=16 bits  ExternalIndexCount=on  PositionUnit=Radians  PositionDataType=single  ParameterInputType=off  CountsPerRevInverseDataType=single
  Speed Measurement : mcbpositiondecoderlib/Speed Measurement  PositionUnit=Radians  PositionScalingDatatype=uint32  SpeedCalculationMode=Time interval for speed calculation  SampleTimeAsync=Ts  MaximumApplicationSpeed=6000  SpeedResolution=5e-6  DelayLength=20  MaximumMeasurableSpeed=-0.98352  MeasurableSpeedResolution=7.6757e-12  SpeedUnit=Radians/Sec  PerUnitSpeed=PU_System.N_base  SpeedDataType=single
  Terminator : Terminator  Commented=on
  The : Gain  OutDataTypeStr=single  RndMeth=Simplest
  ePWM8 : c2802xlib/ePWM  Commented=on  PwmType=C2000_Type4  useModule=ePWM4  ePWMxLINKTBPRD=Not Linked  periodUnits=Clock cycles  timerSource=Specify via dialog  timerPeriod_clk=PWM_Counter_PeriodVel+1  timerPeriod_sec=0.0001  tbshadow=Counter equals to zero  countingMode=Up-Down  phaseActiveEnable=Disable  phaseDirection=Count down after sync  phaseActive=0  synchronizationEnable=off  dcaevt1Sync=off  dcbevt1Sync=off  synchronizationOption=Counter equals to zero (CTR=Zero)  dcbevt1SyncOut=off  dcaevt1SyncOut=off  cmpdSyncOut=off  cmpcSyncOut=off  cmpbSyncOut=off  zeroSyncOut=on  swfSyncOut=off  perSynchronizationOption=Counter equals to period (CTR=PRD)  clockPrescale=1  HSclockPrescale=1  enswap=off  ePWMxAStatus=on  ePWMxAactionLogic1=Do nothing  ePWMxAactionLogic2=Do nothing  ePWMxAactionLogic3=Clear  ePWMxAactionLogic4=Set  ePWMxAactionLogic5=Do nothing  ePWMxAactionLogic6=Do nothing  ePWMxACSFenable=off  ePWMxACSFvalue=Forcing disable  ePWMxASFreload=Zero  ePWMxBStatus=off  ePWMxBactionLogic1=Set  ePWMxBactionLogic2=Clear  ePWMxBactionLogic3=Do nothing  ePWMxBactionLogic4=Do nothing  ePWMxBactionLogic5=Clear  ePWMxBactionLogic6=Set  ePWMxBCSFenable=off  ePWMxBCSFvalue=Forcing disable  ePWMxBSFreload=Zero  ePWNxBOutWay=off  ePWMxLINKCMPA=Not Linked  CMPAUnits=Clock cycles  CMPASource=Input port  CMPAValue_per=50  CMPAValue_clk=floor(PWM_Counter_PeriodVel/2+1)  enCMPAshadow=Counter equals to zero (CTR=Zero)  ePWMxLINKCMPB=Not Linked  CMPBUnits=Clock cycles  CMPBSource=Specify via dialog  CMPBValue_per=50  CMPBValue_clk=floor(PWM_Counter_PeriodVel/2+1)  enCMPBshadow=Counter equals to zero (CTR=Zero)  ePWMxLINKCMPC=Not Linked  CMPCUnits=Clock cycles  CMPCSource=Specify via dialog  CMPCValue_per=50  CMPCValue_clk=32000  enCMPCshadow=Counter equals to zero (CTR=Zero)  ePWMxLINKCMPD=Not Linked  CMPDUnits=Clock cycles  CMPDSource=Specify via dialog  CMPDValue_per=50  CMPDValue_clk=32000  enCMPDshadow=Counter equals to zero (CTR=Zero)  enableDBePWMxA=on  enableDBePWMxB=on  enhalfcycle=off  DBpolarity=Active high complementary (AHC)  DBedgeDelay=Positive  DBSource_ePWMxA=ePWMxA  DBSource_ePWMxB=ePWMxA  DBPeriodUnits=Clock cycles  DBperiodSource=Specify via dialog  REDperiod=15  FEDperiod=15  REDperiod_sec=0  FEDperiod_sec=0  LoadModeDBRED=Immediate without using shadow  LoadModeDBFED=Immediate without using shadow  adcstartModuleA=on  adcrequestEventA=First event  adcstartEventA=Digital Compare Module A Event 1 start of conversion (DCAEVT1.soc)  adcstartEventA_type2=Counter equals to period (CTR=PRD)  adcstartModuleB=off  adcrequestEventB=First event  adcstartEventB=Counter equals to zero (CTR=Zero)  adcstartEventB_type2=Counter equals to zero (CTR=Zero)  intEn=off  intPrd=First event  intSel=Counter equals to zero (CTR=Zero)  intSel_type2=Counter equals to zero (CTR=Zero)  hrpe=off  enHRPWM=off  HRPWM_LoadMode=Counter equals to period (CTR=PRD)  HRPWM_CTLMode=Duty or Period control mode  HRPWM_EDGMode=Both edge  hrpeb=off  enHRPWMB=off  HRPWM_LoadModeB=Counter equals to zero (CTR=ZERO)  HRPWM_CTLModeB=Duty or Period control mode  HRPWM_EDGModeB=Both edge  enHRDBRED=off  enHRDBFED=off  enSFO=on  enautoconv=on  chopperEnable=off  chopperFrequency=1  chopperFirstwidth=1  chopperDuty=12.5%  tripZonesource=Specify via dialog  tzselOSHT1=off  tzselOSHT2=off  tzselOSHT3=off  tzselOSHT4=off  tzselOSHT5=off  tzselOSHT6=off  tzselOSHDCAEV1=off  tzselOSHDCBEV1=off  tzselCBC1=off  tzselCBC2=off  tzselCBC3=off  tzselCBC4=off  tzselCBC5=off  tzselCBC6=off  tzselCBCDCAEV2=off  tzselCBCDCBEV2=off  enTzOstIntr=off  enTzCbcIntr=off  enTzDCAEVT1Intr=off  enTzDCAEVT2Intr=off  enTzDCBEVT1Intr=off  enTzDCBEVT2Intr=off  tzclrCBCLatch=Counter equals to zero (CTR=Zero)  ePWMxAforced=No action  ePWMxBforced=No action  DCAEVT1forced=No action  DCBEVT1forced=No action  DCAEVT2forced=No action  DCBEVT2forced=No action  dcah=Trip Zone 1 input (TZ1)  dcal=Trip Zone 2 input (TZ2)  dcbh=Trip Zone 1 input (TZ1)  dcbl=Trip Zone 2 input (TZ2)  dcah_type2=GPTRIP1SEL/(TZ1)  dcal_type2=GPTRIP2SEL/(TZ2)  dcbh_type2=GPTRIP1SEL/(TZ1)  dcbl_type2=GPTRIP2SEL/(TZ2)  gendcaevt1=Event disabled  gendcaevt2=Event disabled  gendcbevt1=Event disabled  gendcbevt2=Event disabled  dcaevt1src=DCAEVT1 with sync  dcaevt2src=DCAEVT2 with sync  dcbevt1src=DCBEVT1 with sync  dcbevt2src=DCBEVT2 with sync  pulsesel=Counter equals to zero (CTR=Zero)  blankinv=off  blankoffset=0  blankwidth=0  evsrcsel=Filtered version of DCAEVT1 (DCAEVT1FILT)  encape=off
  eQEP : c280xlib/eQEP  useModule=eQEP1  pcInputmode=Quadrature-count  externalClockrate=2x resolution: Count the rising/falling edge  swapPolarityselection=Counterclockwise  qdfOutputport=off  qapPolarityselection=on  qbpPolarityselection=on  qipPolarityselection=on  qspPolarityselection=off  igatePolarityselection=off  sampleTime=-1  pcOutputport=on  pcMaximumvalue=2^16-1  indexInitializationcheck=off  indexInitializationevent=Rising edge  strobeInitializationcheck=off  strobeInitializationevent=Rising edge  softwareInitializationcheck=off  softwareInitializationsource=Set to init value at start up  softwareInitializationmode=on  pcInitialvalue=2147483648  pcResetmode=Reset on the first index event  ieloutputport=on  indexEventlatch=Rising edge  seloutputport=off  strobeEventlatch=Rising edge  pcefOutputport=off  enableEqepcapture=off  qctmrOutputport=off  qcprdOutputport=off  captureTimerprescaler=128  upEventprescaler=128  overflowErrorflag=off  directionErrorflag=off  captureTimerposition=On position counter read  unitTimerperiod=100000000  captureTimerlatch=off  capturePeriodlatch=off  positionCounterlatch=off  soenPolarityselection=off  spselPolarityselection=Index pin is used for sync output  compareValuesource=Specify via dialog  shadowMode=Load on QPOSCNT=0  compareValue=4294967295  syncOutputwidth=1  polaritySyncoutput=Active high  watchdogEnable=off  watchdogTimer=65535  outport1Datatype=auto  outport2Datatype=auto  outport3Datatype=auto  outport4Datatype=auto  outport5Datatype=auto  outport6Datatype=auto  outport7Datatype=auto  outport8Datatype=auto  outport9Datatype=auto  outport10Datatype=auto  outport11Datatype=auto  outport12Datatype=auto  eqepinterrupt_pce=off  eqepinterrupt_qpe=off  eqepinterrupt_qdc=off  eqepinterrupt_wto=off  eqepinterrupt_pcu=off  eqepinterrupt_pco=off  eqepinterrupt_pcr=off  eqepinterrupt_pcm=off  eqepinterrupt_sel=off  eqepinterrupt_iel=off  eqepinterrupt_uto=off  pheOutputport=off  watchdogOutputport=off  outport13Datatype=auto  outport14Datatype=auto
  stop1 : Constant  Commented=on  Value=target.PWM_Counter_Period*0.5  OutDataTypeStr=uint16
  stop2 : Constant  Commented=on  Value=PWM_Counter_PeriodVel*0.5  OutDataTypeStr=uint16
  ThetaE : Outport
  speedfb : Outport  Port=2  VectorParamsAs1DForOutWhenUnconnected=off
  ThetaMec : Outport  Port=3
  wires:
  Speed Measurement/1 -> IIR Filter/1
  IndexFinder/1(EnClosedLoop) -> Data Store Write/1, Delay/1
  Quadrature Decoder/1 -> ThetaMec/1, Mechanical to Electrical Position/1, Speed Measurement/1
  Mechanical to Electrical Position/1 -> The/1
  eQEP/2 -> IndexFinder/1(In1), Quadrature Decoder/2
  NOT/1 -> IndexFinder/Enable
  eQEP/1 -> Quadrature Decoder/1
  Delay/1 -> NOT/1
  The/1 -> ThetaE/1
  stop1/1 -> ePWM8/1
  ADC_C2/1 -> Terminator/1
  IIR Filter/1 -> speedfb/1
  Constant4/1 -> Mechanical to Electrical Position/2

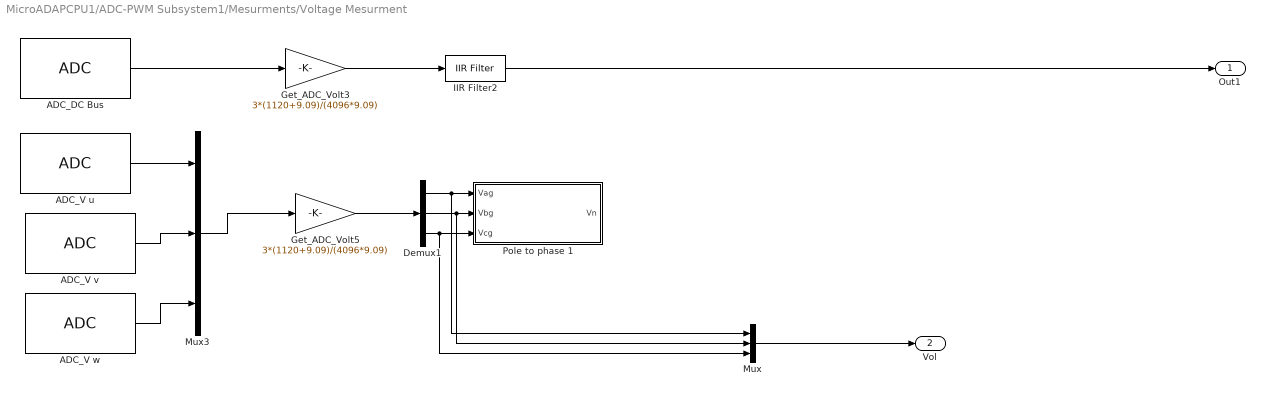
== system MicroADAPCPU1/ADC-PWM Subsystem1/Mesurments/Voltage Mesurment ==
  ADC_DC Bus : c2802xlib/ADC  blkParamProc=C2000_Type4  ADCModule=A  samplingMode=Single sample mode  ADCResolution=12-bit (Single-ended input)  useSOC1=SOC2  useSOC2=SOC0_SOC1  SOCAcquisitionWindow=15  SOCTriggerSource=ePWM1_ADCSOCA  SOCInterruptTrigger=No ADCINT  Ts=-1  dType=uint16  postInterrupt=off  interruptSel=ADCINT1  ADCINTContinuous=on  endma=off  chdma=1  conv1=ADCINA0  conv2=ADCINA0 and ADCINB0  conv1_Type4=ADCIN15  conv2_Type4=ADCIN0 and ADCIN1
  ADC_V u : c2802xlib/ADC  blkParamProc=C2000_Type4  ADCModule=D  samplingMode=Single sample mode  ADCResolution=12-bit (Single-ended input)  useSOC1=SOC0  useSOC2=SOC0_SOC1  SOCAcquisitionWindow=15  SOCTriggerSource=ePWM1_ADCSOCA  SOCInterruptTrigger=No ADCINT  Ts=-1  dType=uint16  postInterrupt=off  interruptSel=ADCINT1  ADCINTContinuous=on  endma=off  chdma=1  conv1=ADCINA0  conv2=ADCINA0 and ADCINB0  conv1_Type4=ADCIN1  conv2_Type4=ADCIN0 and ADCIN1
  ADC_V v : c2802xlib/ADC  blkParamProc=C2000_Type4  ADCModule=D  samplingMode=Single sample mode  ADCResolution=12-bit (Single-ended input)  useSOC1=SOC1  useSOC2=SOC0_SOC1  SOCAcquisitionWindow=15  SOCTriggerSource=ePWM1_ADCSOCA  SOCInterruptTrigger=No ADCINT  Ts=-1  dType=uint16  postInterrupt=off  interruptSel=ADCINT1  ADCINTContinuous=on  endma=off  chdma=1  conv1=ADCINA0  conv2=ADCINA0 and ADCINB0  conv1_Type4=ADCIN0  conv2_Type4=ADCIN0 and ADCIN1
  ADC_V w : c2802xlib/ADC  blkParamProc=C2000_Type4  ADCModule=B  samplingMode=Single sample mode  ADCResolution=12-bit (Single-ended input)  useSOC1=SOC2  useSOC2=SOC0_SOC1  SOCAcquisitionWindow=15  SOCTriggerSource=ePWM1_ADCSOCA  SOCInterruptTrigger=No ADCINT  Ts=-1  dType=uint16  postInterrupt=off  interruptSel=ADCINT1  ADCINTContinuous=on  endma=off  chdma=1  conv1=ADCINA0  conv2=ADCINA0 and ADCINB0  conv1_Type4=ADCIN4  conv2_Type4=ADCIN0 and ADCIN1
  Demux1 : Demux  Outputs=3
  Get_ADC_Volt3 : Gain  Gain=3*(1120+9.09)/(4096*9.09)  OutDataTypeStr=single  RndMeth=Simplest
  Get_ADC_Volt5 : Gain  Gain=3*(1120+9.09)/(4096*9.09)  OutDataTypeStr=single  RndMeth=Simplest
  IIR Filter2 : mcbcontrolslib/IIR Filter  VariantControl=Low Pass Filter  VariantSelect=Low-pass  FilterConstantInputType=Specify via dialog  Filter_constant=0.005  advancedSettings=off  Ts=10e-6  cutOff_freq=79.9774
  Mux : Mux  Inputs=3
  Mux3 : Mux  Inputs=3
  Pole to phase 1 : MATLAB Function  TreatAsAtomicUnit=on
  Out1 : Outport
  Vol : Outport  Port=2
  wires:
  ADC_V v/1 -> Mux3/2
  Mux3/1 -> Get_ADC_Volt5/1
  ADC_V u/1 -> Mux3/1
  Demux1/3 -> Mux/3, Pole to phase 1/3(Vcg)
  Demux1/2 -> Mux/2, Pole to phase 1/2(Vbg)
  Get_ADC_Volt5/1 -> Demux1/1
  Demux1/1 -> Mux/1, Pole to phase 1/1(Vag)
  IIR Filter2/1 -> Out1/1
  ADC_V w/1 -> Mux3/3
  Get_ADC_Volt3/1 -> IIR Filter2/1
  ADC_DC Bus/1 -> Get_ADC_Volt3/1
  Mux/1 -> Vol/1

== system MicroADAPCPU1/Comms/Comms/SCI (Serial Comunication) ==
  In1 : Inport
  Byte Pack : svdutilitieslib/Byte Pack  maskPackedDataType=uint32  datatypes={'single'}  byteAlign=4  blockPlatform=tic2000
  Data_Logging : Subsystem
  Demux2 : Demux  Outputs=2
  While Iterator Subsystem : Subsystem  TreatAsAtomicUnit=on
  wires:
  Demux2/2 -> While Iterator Subsystem/2(Iteration)  "SCI_Tx_Iteration"
  Demux2/1 -> While Iterator Subsystem/1(Data)  "SCI_Tx_Data"
  In1/1 -> Byte Pack/1
  Data_Logging/1(SCI_Tx) -> Demux2/1
  Byte Pack/1 -> Data_Logging/1(Data_Log)

== system MicroADAPCPU1/Comms/SCI (Code Generation) 40khz/Data_Logging ==
  note: Fast Serial Data Monitoring (32-bit)
  Data_Log : Inport
  Counter Limited : simulink/Sources/Counter Limited  uplimit=1200-1  tsamp=-1
  Data : Subsystem  TreatAsAtomicUnit=on
  End : Subsystem  TreatAsAtomicUnit=on
  If : If  IfExpression=u1 == 0  ElseIfExpressions=u1 == 1200
  Merge : Merge  Inputs=3
  Merge1 : Merge  Inputs=3
  Mux : Mux  Inputs=2
  Start : Subsystem  TreatAsAtomicUnit=on
  Width : Width  OutDataTypeMode=All ports same datatype  DataType=uint16
  SCI_Tx : Outport
  wires:
  Data_Log/1 -> Data/1(Data), End/1(Data), Start/1(Data), Width/1
  Mux/1 -> SCI_Tx/1
  Data/2(Iteration) -> Merge1/3
  End/2(Iteration) -> Merge1/2
  End/1(Data_out) -> Merge/2
  If/1 -> Start/Action
  Merge1/1 -> Mux/2  "SCI_Tx_Iteration"
  If/2 -> End/Action
  Start/1(Data_out) -> Merge/1
  Start/2(Iteration) -> Merge1/1
  Counter Limited/1 -> If/1
  Merge/1 -> Mux/1  "SCI_Tx_Data"
  Width/1 -> Start/2(Data_width), End/2(Data_width), Data/2(Data_width)
  Data/1(Data_out) -> Merge/3
  If/3 -> Data/Action
